simulink model "stepper_sim"  (R2015a)
settings: Solver=FixedStepDiscrete  StartTime=0.0  StopTime=240  FixedStep=0.1  RelTol=1e-3
libraries: arduino_io_lib x3, simulink x2
settings Model: Creator=gcampa  LastModifiedBy=Osman
settings DataIOCC: SignalLoggingSaveFormat=ModelDataLogs
settings OptimizationCC: ExpressionDepthLimit=2147483647
settings DebuggingCC: UnderspecifiedInitializationDetection=Classic  MergeDetectMultiDrivingBlocksExec=none  SolverPrmCheckMsg=warning  FcnCallInpInsideContextMsg=UseLocalSettings  StateNameClashWarn=warning
settings GRTTargetCC: CombineOutputUpdateFcns=off  GRTInterface=on

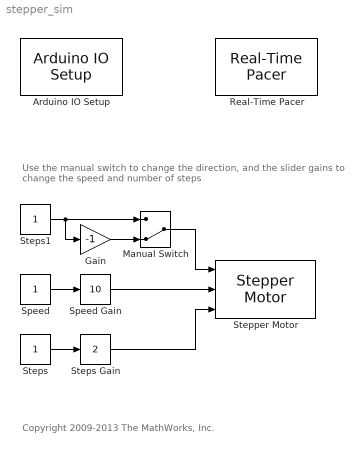
== system stepper_sim ==
  note: Use the manual switch to change the direction,
      | and the slider gains to change the speed and number of steps
  note: Copyright 2009-2013 The MathWorks, Inc.
  Arduino IO Setup : arduino_io_lib/Arduino IO Setup  Priority=3  arduinoVar=Temporary arduino variable: Arduino1  workspaceVarName=a  comPort=COM9
  Gain : Gain  Gain=-1
  Manual Switch : ManualSwitch  CurrentSetting=0
  Real-Time Pacer : arduino_io_lib/Real-Time Pacer  simTimePerRealTime=1
  Speed : Constant
  Speed Gain : simulink/Math Operations/Slider Gain  low=0  gain=10  high=60
  Stepper Motor : arduino_io_lib/Stepper Motor  arduinoVar=Temporary arduino variable: Arduino1  motorNum=1  motionStyle=single  sendOnChange=on  T=0.1
  Steps : Constant
  Steps Gain : simulink/Math Operations/Slider Gain  low=0  gain=2  high=10
  Steps1 : Constant
  wires:
  Steps/1 -> Steps Gain/1
  Speed/1 -> Speed Gain/1
  Manual Switch/1 -> Stepper Motor/1
  Steps1/1 -> Manual Switch/1, Gain/1
  Gain/1 -> Manual Switch/2
  Steps Gain/1 -> Stepper Motor/3
  Speed Gain/1 -> Stepper Motor/2
